simulink model "observerModel_MS"  (R2022b)
settings: Solver=ode15s  StartTime=0.0  StopTime=duration  MaxStep=0.02  RelTol=0.02  AbsTol=0.02  EnableMultiTasking=on
values from neighbouring files (symbols this model uses):
  beta1 = s(8)    [RunObserver.m]
  beta2 = s(7)    [RunObserver.m]
  delta_t = time(2) - time (1)    [RunObserver.m]
  df = 1    [RunObserver.m]
  f_oto = 2    [RunObserver.m]
  f_scc = 2    [RunObserver.m]
  f_visO = 0.2    [RunObserver.m]
  f_visV = 2    [RunObserver.m]
  f_visX = 2    [RunObserver.m]
  G0 = [0 0 -ground_truth]'    [RunObserver.m]
  GG0 = [0 0 -hypo]'    [RunObserver.m]
  kaa = -.5*[1 1 1]'    [RunObserver.m]
  Kea = s(1)^(1/2)*[1 1 1]    [RunObserver.m]
  Kef = s(3)^(1/2)*[1 1 1]    [RunObserver.m]
  Kew = s(2)^(1/2)*[1 1 1]    [RunObserver.m]
  Kfast = s(4)    [RunObserver.m]
  kfg = 4*[1 1 1]'    [RunObserver.m]
  kfw = 8*[1 1 1]'    [RunObserver.m]
  kgvg = 5*[1 1 1]'    [RunObserver.m]
  kwg = 1*[1 1 1]'    [RunObserver.m]
  kwvw = 10*[1 1 1]'    [RunObserver.m]
  kww = 8*[1 1 1]'    [RunObserver.m]
  kxdotva = 0.75*[1 1 1]'    [RunObserver.m]
  kxvv = 0.1*[1 1 1]'    [RunObserver.m]
  ms_exp = s(6)    [RunObserver.m]
  oto_a = 60*[1 1 1]'    [RunObserver.m]
  oto_Ka = 1.3*[1 1 1]'    [RunObserver.m]
  Q0 = [cos(E_angle/2) E(1)*sin(E_angle/2) E(2)*sin(E_angle/2) E(3)*sin(E_angle/2)]'    [RunObserver.m]
  tau_a = tau_a_value*[1 1 1]'    [RunObserver.m]
  tau_scc = tau_scc_value*[1 1 1]'    [RunObserver.m]
  x_leak = 0.6    [RunObserver.m]
  y_leak = 0.6    [RunObserver.m]
  z_leak = 10    [RunObserver.m]
(part 3 of 3)

== system observerModel_MS/Quaternion Rotator2/Head to Limbic Angular Velocity Transform Rotation Matrix/Quaternion to Direction Cosine1/A33 ==
  q : Inport
  Demux : Demux
  Product{,1..3} (4 alike) : Product  RndMeth=Zero
  Sum : Sum  Inputs=+--+
  A33 : Outport
  wires:
  Demux/1 -> Product/1, Product/2
  Demux/2 -> Product1/1, Product1/2
  Demux/3 -> Product2/1, Product2/2
  Demux/4 -> Product3/1, Product3/2
  Product/1 -> Sum/1
  Product1/1 -> Sum/2
  Product2/1 -> Sum/3
  Product3/1 -> Sum/4
  q/1 -> Demux/1
  Sum/1 -> A33/1

== system observerModel_MS/Quaternion Rotator2/Quaternion Integrator/delta_q/C ==
  omega : Inport
  q : Inport  Port=2
  C1 : Subsystem
  C2 : Subsystem
  C3 : Subsystem
  C4 : Subsystem
  Mux : Mux
  C : Outport
  wires:
  omega/1 -> C1/1(omega), C2/1(omega), C3/1(omega), C4/1(omega)
  q/1 -> C4/2(q), C3/2(q), C2/2(q), C1/2(q)
  C1/1(c1) -> Mux/1
  C2/1(c2) -> Mux/2
  C3/1(c3) -> Mux/3
  C4/1(c4) -> Mux/4
  Mux/1 -> C/1

== system observerModel_MS/Quaternion Rotator2/Quaternion Integrator/delta_q/K ==
  Product : Product  RndMeth=Zero
  k : Constant  Value=1/delta_t
  value : Constant  Value=0.9
  K : Outport
  wires:
  k/1 -> Product/1
  Product/1 -> K/1
  value/1 -> Product/2

== system observerModel_MS/Quaternion Rotator2/Quaternion Integrator/delta_q/Z ==
  q : Inport
  Constant : Constant
  Demux : Demux
  Product{,1..3} (4 alike) : Product  RndMeth=Zero
  Sum : Sum  Inputs=++++
  Sum1 : Sum  Inputs=+-
  z : Outport
  wires:
  Demux/1 -> Product/1, Product/2
  Demux/2 -> Product1/1, Product1/2
  Demux/3 -> Product2/1, Product2/2
  Demux/4 -> Product3/1, Product3/2
  q/1 -> Demux/1
  Product/1 -> Sum/1
  Product1/1 -> Sum/2
  Product2/1 -> Sum/3
  Product3/1 -> Sum/4
  Sum/1 -> Sum1/2
  Constant/1 -> Sum1/1
  Sum1/1 -> z/1

== system observerModel_MS/Quaternion Rotator2/Rotation/Azimuthal Integrator/Matrix Multiplication1 ==
  D_Cos : Inport
  omega_rad : Inport  Port=2
  Demux : Demux  Outputs=3
      settings: DisplayOption=none
  Mux : Mux  Inputs=3
  Product : Product  Multiplication=Matrix(*)  RndMeth=Zero
  omega_rad' : Outport
  wires:
  Product/1 -> Demux/1
  Demux/1 -> Mux/1
  Demux/2 -> Mux/2
  Demux/3 -> Mux/3
  D_Cos/1 -> Product/1
  Mux/1 -> omega_rad'/1
  omega_rad/1 -> Product/2

== system observerModel_MS/Quaternion Rotator/Head to Limbic Angular Velocity Transform/Quaternion Integrator1/delta_q/C ==
  omega : Inport
  q : Inport  Port=2
  C1 : Subsystem
  C2 : Subsystem
  C3 : Subsystem
  C4 : Subsystem
  Mux : Mux
  C : Outport
  wires:
  omega/1 -> C1/1(omega), C2/1(omega), C3/1(omega), C4/1(omega)
  q/1 -> C4/2(q), C3/2(q), C2/2(q), C1/2(q)
  C1/1(c1) -> Mux/1
  C2/1(c2) -> Mux/2
  C3/1(c3) -> Mux/3
  C4/1(c4) -> Mux/4
  Mux/1 -> C/1

== system observerModel_MS/Quaternion Rotator/Head to Limbic Angular Velocity Transform/Quaternion Integrator1/delta_q/K ==
  Product : Product  RndMeth=Zero
  k : Constant  Value=1/delta_t
  value : Constant  Value=0.9
  K : Outport
  wires:
  k/1 -> Product/1
  Product/1 -> K/1
  value/1 -> Product/2

== system observerModel_MS/Quaternion Rotator/Head to Limbic Angular Velocity Transform/Quaternion Integrator1/delta_q/Z ==
  q : Inport
  Constant : Constant
  Demux : Demux
  Product{,1..3} (4 alike) : Product  RndMeth=Zero
  Sum : Sum  Inputs=++++
  Sum1 : Sum  Inputs=+-
  z : Outport
  wires:
  Demux/1 -> Product/1, Product/2
  Demux/2 -> Product1/1, Product1/2
  Demux/3 -> Product2/1, Product2/2
  Demux/4 -> Product3/1, Product3/2
  q/1 -> Demux/1
  Product/1 -> Sum/1
  Product1/1 -> Sum/2
  Product2/1 -> Sum/3
  Product3/1 -> Sum/4
  Sum/1 -> Sum1/2
  Constant/1 -> Sum1/1
  Sum1/1 -> z/1

== system observerModel_MS/Quaternion Rotator/Quaternion Integrator/delta_q/C/C1 ==
  omega : Inport
  q : Inport  Port=2
  Demux : Demux  Outputs=3
  Demux1 : Demux
  Gain : Gain  Gain=-0.5
  Product : Product  RndMeth=Zero
  Product1 : Product  RndMeth=Zero
  Product2 : Product  RndMeth=Zero
  Sum : Sum  Inputs=+++
  Terminator : Terminator
  c1 : Outport
  wires:
  Demux1/2 -> Product/2
  Demux/1 -> Product/1
  Demux1/3 -> Product1/2
  Demux/2 -> Product1/1
  Demux1/4 -> Product2/2
  Demux/3 -> Product2/1
  Product/1 -> Sum/1
  Product1/1 -> Sum/2
  Product2/1 -> Sum/3
  Sum/1 -> Gain/1
  omega/1 -> Demux/1
  Gain/1 -> c1/1
  q/1 -> Demux1/1
  Demux1/1 -> Terminator/1

== system observerModel_MS/Quaternion Rotator/Quaternion Integrator/delta_q/C/C2 ==
  omega : Inport
  q : Inport  Port=2
  Demux : Demux  Outputs=3
  Demux1 : Demux
  Gain : Gain  Gain=0.5
  Product : Product  RndMeth=Zero
  Product1 : Product  RndMeth=Zero
  Product2 : Product  RndMeth=Zero
  Sum : Sum  Inputs=++-
  Terminator : Terminator
  c2 : Outport
  wires:
  Product/1 -> Sum/1
  Product1/1 -> Sum/2
  Product2/1 -> Sum/3
  Sum/1 -> Gain/1
  omega/1 -> Demux/1
  Gain/1 -> c2/1
  q/1 -> Demux1/1
  Demux1/1 -> Product/2
  Demux/1 -> Product/1
  Demux1/3 -> Product1/2
  Demux/3 -> Product1/1
  Demux1/4 -> Product2/2
  Demux/2 -> Product2/1
  Demux1/2 -> Terminator/1

== system observerModel_MS/Quaternion Rotator/Quaternion Integrator/delta_q/C/C3 ==
  omega : Inport
  q : Inport  Port=2
  Demux : Demux  Outputs=3
  Demux1 : Demux
  Gain : Gain  Gain=0.5
  Product : Product  RndMeth=Zero
  Product1 : Product  RndMeth=Zero
  Product2 : Product  RndMeth=Zero
  Sum : Sum  Inputs=++-
  Terminator : Terminator
  c3 : Outport
  wires:
  Product/1 -> Sum/1
  Product1/1 -> Sum/2
  Product2/1 -> Sum/3
  Sum/1 -> Gain/1
  omega/1 -> Demux/1
  Gain/1 -> c3/1
  q/1 -> Demux1/1
  Demux1/1 -> Product/2
  Demux/2 -> Product/1
  Demux1/4 -> Product1/2
  Demux/1 -> Product1/1
  Demux1/2 -> Product2/2
  Demux/3 -> Product2/1
  Demux1/3 -> Terminator/1

== system observerModel_MS/Quaternion Rotator/Quaternion Integrator/delta_q/C/C4 ==
  omega : Inport
  q : Inport  Port=2
  Demux : Demux  Outputs=3
  Demux1 : Demux
  Gain : Gain  Gain=0.5
  Product : Product  RndMeth=Zero
  Product1 : Product  RndMeth=Zero
  Product2 : Product  RndMeth=Zero
  Sum : Sum  Inputs=++-
  Terminator : Terminator
  c4 : Outport
  wires:
  Product/1 -> Sum/1
  Product1/1 -> Sum/2
  Product2/1 -> Sum/3
  Sum/1 -> Gain/1
  omega/1 -> Demux/1
  Gain/1 -> c4/1
  q/1 -> Demux1/1
  Demux1/1 -> Product/2
  Demux/3 -> Product/1
  Demux1/2 -> Product1/2
  Demux/2 -> Product1/1
  Demux1/3 -> Product2/2
  Demux/1 -> Product2/1
  Demux1/4 -> Terminator/1

== system observerModel_MS/Quaternion Rotator2/Head to Limbic Angular Velocity Transform Rotation Matrix/Quaternion Integrator1/delta_q/C ==
  omega : Inport
  q : Inport  Port=2
  C1 : Subsystem
  C2 : Subsystem
  C3 : Subsystem
  C4 : Subsystem
  Mux : Mux
  C : Outport
  wires:
  omega/1 -> C1/1(omega), C2/1(omega), C3/1(omega), C4/1(omega)
  q/1 -> C4/2(q), C3/2(q), C2/2(q), C1/2(q)
  C1/1(c1) -> Mux/1
  C2/1(c2) -> Mux/2
  C3/1(c3) -> Mux/3
  C4/1(c4) -> Mux/4
  Mux/1 -> C/1

== system observerModel_MS/Quaternion Rotator2/Head to Limbic Angular Velocity Transform Rotation Matrix/Quaternion Integrator1/delta_q/K ==
  Product : Product  RndMeth=Zero
  k : Constant  Value=1/delta_t
  value : Constant  Value=0.9
  K : Outport
  wires:
  k/1 -> Product/1
  Product/1 -> K/1
  value/1 -> Product/2

== system observerModel_MS/Quaternion Rotator2/Head to Limbic Angular Velocity Transform Rotation Matrix/Quaternion Integrator1/delta_q/Z ==
  q : Inport
  Constant : Constant
  Demux : Demux
  Product{,1..3} (4 alike) : Product  RndMeth=Zero
  Sum : Sum  Inputs=++++
  Sum1 : Sum  Inputs=+-
  z : Outport
  wires:
  Demux/1 -> Product/1, Product/2
  Demux/2 -> Product1/1, Product1/2
  Demux/3 -> Product2/1, Product2/2
  Demux/4 -> Product3/1, Product3/2
  q/1 -> Demux/1
  Product/1 -> Sum/1
  Product1/1 -> Sum/2
  Product2/1 -> Sum/3
  Product3/1 -> Sum/4
  Sum/1 -> Sum1/2
  Constant/1 -> Sum1/1
  Sum1/1 -> z/1

== system observerModel_MS/Quaternion Rotator2/Quaternion Integrator/delta_q/C/C1 ==
  omega : Inport
  q : Inport  Port=2
  Demux : Demux  Outputs=3
  Demux1 : Demux
  Gain : Gain  Gain=-0.5
  Product : Product  RndMeth=Zero
  Product1 : Product  RndMeth=Zero
  Product2 : Product  RndMeth=Zero
  Sum : Sum  Inputs=+++
  Terminator : Terminator
  c1 : Outport
  wires:
  Demux1/2 -> Product/2
  Demux/1 -> Product/1
  Demux1/3 -> Product1/2
  Demux/2 -> Product1/1
  Demux1/4 -> Product2/2
  Demux/3 -> Product2/1
  Product/1 -> Sum/1
  Product1/1 -> Sum/2
  Product2/1 -> Sum/3
  Sum/1 -> Gain/1
  omega/1 -> Demux/1
  Gain/1 -> c1/1
  q/1 -> Demux1/1
  Demux1/1 -> Terminator/1

== system observerModel_MS/Quaternion Rotator2/Quaternion Integrator/delta_q/C/C2 ==
  omega : Inport
  q : Inport  Port=2
  Demux : Demux  Outputs=3
  Demux1 : Demux
  Gain : Gain  Gain=0.5
  Product : Product  RndMeth=Zero
  Product1 : Product  RndMeth=Zero
  Product2 : Product  RndMeth=Zero
  Sum : Sum  Inputs=++-
  Terminator : Terminator
  c2 : Outport
  wires:
  Product/1 -> Sum/1
  Product1/1 -> Sum/2
  Product2/1 -> Sum/3
  Sum/1 -> Gain/1
  omega/1 -> Demux/1
  Gain/1 -> c2/1
  q/1 -> Demux1/1
  Demux1/1 -> Product/2
  Demux/1 -> Product/1
  Demux1/3 -> Product1/2
  Demux/3 -> Product1/1
  Demux1/4 -> Product2/2
  Demux/2 -> Product2/1
  Demux1/2 -> Terminator/1

== system observerModel_MS/Quaternion Rotator2/Quaternion Integrator/delta_q/C/C3 ==
  omega : Inport
  q : Inport  Port=2
  Demux : Demux  Outputs=3
  Demux1 : Demux
  Gain : Gain  Gain=0.5
  Product : Product  RndMeth=Zero
  Product1 : Product  RndMeth=Zero
  Product2 : Product  RndMeth=Zero
  Sum : Sum  Inputs=++-
  Terminator : Terminator
  c3 : Outport
  wires:
  Product/1 -> Sum/1
  Product1/1 -> Sum/2
  Product2/1 -> Sum/3
  Sum/1 -> Gain/1
  omega/1 -> Demux/1
  Gain/1 -> c3/1
  q/1 -> Demux1/1
  Demux1/1 -> Product/2
  Demux/2 -> Product/1
  Demux1/4 -> Product1/2
  Demux/1 -> Product1/1
  Demux1/2 -> Product2/2
  Demux/3 -> Product2/1
  Demux1/3 -> Terminator/1

== system observerModel_MS/Quaternion Rotator2/Quaternion Integrator/delta_q/C/C4 ==
  omega : Inport
  q : Inport  Port=2
  Demux : Demux  Outputs=3
  Demux1 : Demux
  Gain : Gain  Gain=0.5
  Product : Product  RndMeth=Zero
  Product1 : Product  RndMeth=Zero
  Product2 : Product  RndMeth=Zero
  Sum : Sum  Inputs=++-
  Terminator : Terminator
  c4 : Outport
  wires:
  Product/1 -> Sum/1
  Product1/1 -> Sum/2
  Product2/1 -> Sum/3
  Sum/1 -> Gain/1
  omega/1 -> Demux/1
  Gain/1 -> c4/1
  q/1 -> Demux1/1
  Demux1/1 -> Product/2
  Demux/3 -> Product/1
  Demux1/2 -> Product1/2
  Demux/2 -> Product1/1
  Demux1/3 -> Product2/2
  Demux/1 -> Product2/1
  Demux1/4 -> Terminator/1

== system observerModel_MS/Quaternion Rotator/Head to Limbic Angular Velocity Transform/Quaternion Integrator1/delta_q/C/C1 ==
  omega : Inport
  q : Inport  Port=2
  Demux : Demux  Outputs=3
  Demux1 : Demux
  Gain : Gain  Gain=-0.5
  Product : Product  RndMeth=Zero
  Product1 : Product  RndMeth=Zero
  Product2 : Product  RndMeth=Zero
  Sum : Sum  Inputs=+++
  Terminator : Terminator
  c1 : Outport
  wires:
  Demux1/2 -> Product/2
  Demux/1 -> Product/1
  Demux1/3 -> Product1/2
  Demux/2 -> Product1/1
  Demux1/4 -> Product2/2
  Demux/3 -> Product2/1
  Product/1 -> Sum/1
  Product1/1 -> Sum/2
  Product2/1 -> Sum/3
  Sum/1 -> Gain/1
  omega/1 -> Demux/1
  Gain/1 -> c1/1
  q/1 -> Demux1/1
  Demux1/1 -> Terminator/1

== system observerModel_MS/Quaternion Rotator/Head to Limbic Angular Velocity Transform/Quaternion Integrator1/delta_q/C/C2 ==
  omega : Inport
  q : Inport  Port=2
  Demux : Demux  Outputs=3
  Demux1 : Demux
  Gain : Gain  Gain=0.5
  Product : Product  RndMeth=Zero
  Product1 : Product  RndMeth=Zero
  Product2 : Product  RndMeth=Zero
  Sum : Sum  Inputs=++-
  Terminator : Terminator
  c2 : Outport
  wires:
  Product/1 -> Sum/1
  Product1/1 -> Sum/2
  Product2/1 -> Sum/3
  Sum/1 -> Gain/1
  omega/1 -> Demux/1
  Gain/1 -> c2/1
  q/1 -> Demux1/1
  Demux1/1 -> Product/2
  Demux/1 -> Product/1
  Demux1/3 -> Product1/2
  Demux/3 -> Product1/1
  Demux1/4 -> Product2/2
  Demux/2 -> Product2/1
  Demux1/2 -> Terminator/1

== system observerModel_MS/Quaternion Rotator/Head to Limbic Angular Velocity Transform/Quaternion Integrator1/delta_q/C/C3 ==
  omega : Inport
  q : Inport  Port=2
  Demux : Demux  Outputs=3
  Demux1 : Demux
  Gain : Gain  Gain=0.5
  Product : Product  RndMeth=Zero
  Product1 : Product  RndMeth=Zero
  Product2 : Product  RndMeth=Zero
  Sum : Sum  Inputs=++-
  Terminator : Terminator
  c3 : Outport
  wires:
  Product/1 -> Sum/1
  Product1/1 -> Sum/2
  Product2/1 -> Sum/3
  Sum/1 -> Gain/1
  omega/1 -> Demux/1
  Gain/1 -> c3/1
  q/1 -> Demux1/1
  Demux1/1 -> Product/2
  Demux/2 -> Product/1
  Demux1/4 -> Product1/2
  Demux/1 -> Product1/1
  Demux1/2 -> Product2/2
  Demux/3 -> Product2/1
  Demux1/3 -> Terminator/1

== system observerModel_MS/Quaternion Rotator/Head to Limbic Angular Velocity Transform/Quaternion Integrator1/delta_q/C/C4 ==
  omega : Inport
  q : Inport  Port=2
  Demux : Demux  Outputs=3
  Demux1 : Demux
  Gain : Gain  Gain=0.5
  Product : Product  RndMeth=Zero
  Product1 : Product  RndMeth=Zero
  Product2 : Product  RndMeth=Zero
  Sum : Sum  Inputs=++-
  Terminator : Terminator
  c4 : Outport
  wires:
  Product/1 -> Sum/1
  Product1/1 -> Sum/2
  Product2/1 -> Sum/3
  Sum/1 -> Gain/1
  omega/1 -> Demux/1
  Gain/1 -> c4/1
  q/1 -> Demux1/1
  Demux1/1 -> Product/2
  Demux/3 -> Product/1
  Demux1/2 -> Product1/2
  Demux/2 -> Product1/1
  Demux1/3 -> Product2/2
  Demux/1 -> Product2/1
  Demux1/4 -> Terminator/1

== system observerModel_MS/Quaternion Rotator2/Head to Limbic Angular Velocity Transform Rotation Matrix/Quaternion Integrator1/delta_q/C/C1 ==
  omega : Inport
  q : Inport  Port=2
  Demux : Demux  Outputs=3
  Demux1 : Demux
  Gain : Gain  Gain=-0.5
  Product : Product  RndMeth=Zero
  Product1 : Product  RndMeth=Zero
  Product2 : Product  RndMeth=Zero
  Sum : Sum  Inputs=+++
  Terminator : Terminator
  c1 : Outport
  wires:
  Demux1/2 -> Product/2
  Demux/1 -> Product/1
  Demux1/3 -> Product1/2
  Demux/2 -> Product1/1
  Demux1/4 -> Product2/2
  Demux/3 -> Product2/1
  Product/1 -> Sum/1
  Product1/1 -> Sum/2
  Product2/1 -> Sum/3
  Sum/1 -> Gain/1
  omega/1 -> Demux/1
  Gain/1 -> c1/1
  q/1 -> Demux1/1
  Demux1/1 -> Terminator/1

== system observerModel_MS/Quaternion Rotator2/Head to Limbic Angular Velocity Transform Rotation Matrix/Quaternion Integrator1/delta_q/C/C2 ==
  omega : Inport
  q : Inport  Port=2
  Demux : Demux  Outputs=3
  Demux1 : Demux
  Gain : Gain  Gain=0.5
  Product : Product  RndMeth=Zero
  Product1 : Product  RndMeth=Zero
  Product2 : Product  RndMeth=Zero
  Sum : Sum  Inputs=++-
  Terminator : Terminator
  c2 : Outport
  wires:
  Product/1 -> Sum/1
  Product1/1 -> Sum/2
  Product2/1 -> Sum/3
  Sum/1 -> Gain/1
  omega/1 -> Demux/1
  Gain/1 -> c2/1
  q/1 -> Demux1/1
  Demux1/1 -> Product/2
  Demux/1 -> Product/1
  Demux1/3 -> Product1/2
  Demux/3 -> Product1/1
  Demux1/4 -> Product2/2
  Demux/2 -> Product2/1
  Demux1/2 -> Terminator/1

== system observerModel_MS/Quaternion Rotator2/Head to Limbic Angular Velocity Transform Rotation Matrix/Quaternion Integrator1/delta_q/C/C3 ==
  omega : Inport
  q : Inport  Port=2
  Demux : Demux  Outputs=3
  Demux1 : Demux
  Gain : Gain  Gain=0.5
  Product : Product  RndMeth=Zero
  Product1 : Product  RndMeth=Zero
  Product2 : Product  RndMeth=Zero
  Sum : Sum  Inputs=++-
  Terminator : Terminator
  c3 : Outport
  wires:
  Product/1 -> Sum/1
  Product1/1 -> Sum/2
  Product2/1 -> Sum/3
  Sum/1 -> Gain/1
  omega/1 -> Demux/1
  Gain/1 -> c3/1
  q/1 -> Demux1/1
  Demux1/1 -> Product/2
  Demux/2 -> Product/1
  Demux1/4 -> Product1/2
  Demux/1 -> Product1/1
  Demux1/2 -> Product2/2
  Demux/3 -> Product2/1
  Demux1/3 -> Terminator/1

== system observerModel_MS/Quaternion Rotator2/Head to Limbic Angular Velocity Transform Rotation Matrix/Quaternion Integrator1/delta_q/C/C4 ==
  omega : Inport
  q : Inport  Port=2
  Demux : Demux  Outputs=3
  Demux1 : Demux
  Gain : Gain  Gain=0.5
  Product : Product  RndMeth=Zero
  Product1 : Product  RndMeth=Zero
  Product2 : Product  RndMeth=Zero
  Sum : Sum  Inputs=++-
  Terminator : Terminator
  c4 : Outport
  wires:
  Product/1 -> Sum/1
  Product1/1 -> Sum/2
  Product2/1 -> Sum/3
  Sum/1 -> Gain/1
  omega/1 -> Demux/1
  Gain/1 -> c4/1
  q/1 -> Demux1/1
  Demux1/1 -> Product/2
  Demux/3 -> Product/1
  Demux1/2 -> Product1/2
  Demux/2 -> Product1/1
  Demux1/3 -> Product2/2
  Demux/1 -> Product2/1
  Demux1/4 -> Terminator/1
